simulink model "rayTrace_th"  (R2018b)
settings: Solver=FixedStepAuto  StartTime=0.0  StopTime=0  FixedStep=1  RelTol=1e-3
values from neighbouring files (symbols this model uses):
  grnd2CamRotMat = calculateRotationMatrix(     camEulAngles_rad(1),camEulAngles_rad(2),camEulAngles_rad(3))    [rayTrace_init.m]    (also in rayTrace_ts1.m = calculateRotationMatrix(     roll_deg*pi/180,pitch_deg*pi/18; rayTrace_ts3.m = calculateRotationMatrix(     roll_deg*pi/180,pitch_deg*pi/18; rayTrace_ts4.m)
  pixelCol = pixelCoords(ii,2)    [rayTrace_ts1.m]    (also in rayTrace_ts2.m; rayTrace_ts4.m = mean([pixCoords(2) pixCoords(4)]))
  pixelRow = pixelCoords(ii,1)    [rayTrace_ts1.m]    (also in rayTrace_ts2.m; rayTrace_ts4.m = mean([pixCoords(1) pixCoords(3)]))
undefined symbols (not defined in the file or in its folder): getVal, rayTrace, rayTrace_ul
settings Model: Creator=mcobb  LastModifiedBy=MAE-NCSUCORE

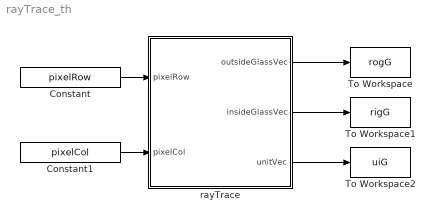
== system rayTrace_th ==
  Constant : Constant  Value=pixelRow
  Constant1 : Constant  Value=pixelCol
  To Workspace : ToWorkspace  VariableName=rogG  SampleTime=-1
  To Workspace1 : ToWorkspace  VariableName=rigG  SampleTime=-1
  To Workspace2 : ToWorkspace  VariableName=uiG  SampleTime=-1
  rayTrace : Subsystem  AncestorBlock=rayTrace_ul/rayTrace  mask{camPosVec_cm=[-30.5 -2 26], camEulAngles_deg=[0 133.9 180.6], dist2Glass_cm=7, indOfRefVec=[1 1 1], glassPlane=1, glassThickness_cm=0.75*2.54, imageDimsVec_px=getVal('sideImageSize_px'), camFOV_deg=getVal('cameraFOV_deg')}
      mask prompts: camPosVec_cm "Camera Position Vector, cm"; camEulAngles_deg "Camera Euler Angles, deg"; dist2Glass_cm "Distance to glass, cm"; indOfRefVec "Indices of refraction [air glass water]"; glassPlane "Glass plane (1 = xy, 2 = xz)"; glassThickness_cm "Glass thickness, cm"; imageDimsVec_px "Image dimensions, px [rows cols]"; camFOV_deg "Camera field of view angles,deg  [horiz vert]"
      mask init:
      | rayTrace_init
  wires:
  Constant/1 -> rayTrace/1(pixelRow)
  Constant1/1 -> rayTrace/2(pixelCol)
  rayTrace/1(outsideGlassVec) -> To Workspace/1
  rayTrace/3(unitVec) -> To Workspace2/1
  rayTrace/2(insideGlassVec) -> To Workspace1/1

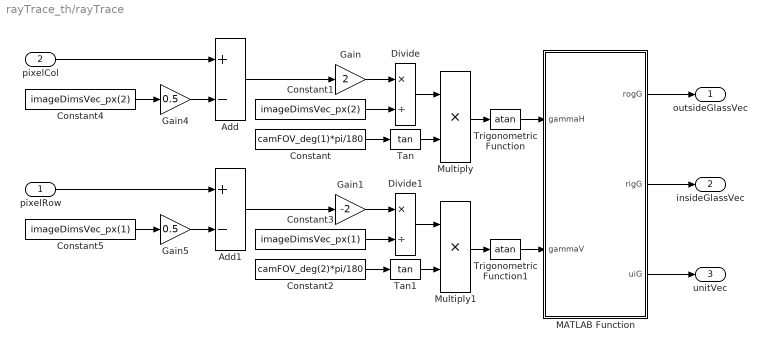
== system rayTrace_th/rayTrace ==
  pixelRow : Inport
  pixelCol : Inport  Port=2
  Add : Sum  Inputs=+-
  Add1 : Sum  Inputs=+-
  Constant : Constant  Value=camFOV_deg(1)*pi/180
  Constant1 : Constant  Value=imageDimsVec_px(2)
  Constant2 : Constant  Value=camFOV_deg(2)*pi/180
  Constant3 : Constant  Value=imageDimsVec_px(1)
  Constant4 : Constant  Value=imageDimsVec_px(2)
  Constant5 : Constant  Value=imageDimsVec_px(1)
  Divide : Product  Inputs=*/
  Divide1 : Product  Inputs=*/
  Gain : Gain  Gain=2
  Gain1 : Gain  Gain=-2
  Gain4 : Gain  Gain=0.5
  Gain5 : Gain  Gain=0.5
  MATLAB Function : MATLAB Function  TreatAsAtomicUnit=on
  Multiply : Product
  Multiply1 : Product
  Tan : Trigonometry  Operator=tan
  Tan1 : Trigonometry  Operator=tan
  Trigonometric Function : Trigonometry  Operator=atan
  Trigonometric Function1 : Trigonometry  Operator=atan
  outsideGlassVec : Outport
  insideGlassVec : Outport  Port=2
  unitVec : Outport  Port=3
  wires:
  Add1/1 -> Gain1/1
  Gain5/1 -> Add1/2
  pixelRow/1 -> Add1/1
  Constant5/1 -> Gain5/1
  Gain4/1 -> Add/2
  Constant4/1 -> Gain4/1
  Add/1 -> Gain/1
  pixelCol/1 -> Add/1
  Divide1/1 -> Multiply1/1
  Tan1/1 -> Multiply1/2
  Multiply1/1 -> Trigonometric Function1/1
  Trigonometric Function1/1 -> MATLAB Function/2(gammaV)
  Constant2/1 -> Tan1/1
  Constant3/1 -> Divide1/2
  Gain1/1 -> Divide1/1
  Constant1/1 -> Divide/2
  Gain/1 -> Divide/1
  Divide/1 -> Multiply/1
  Constant/1 -> Tan/1
  Tan/1 -> Multiply/2
  Multiply/1 -> Trigonometric Function/1
  Trigonometric Function/1 -> MATLAB Function/1(gammaH)
  MATLAB Function/1(rogG) -> outsideGlassVec/1
  MATLAB Function/3(uiG) -> unitVec/1
  MATLAB Function/2(rigG) -> insideGlassVec/1

== matlab function rayTrace_th/rayTrace/MATLAB Function ==
  data: rogG output; gammaH input; gammaV input; rigG output; uiG output; camPosVec_cm parameter; grnd2CamRotMat parameter; dist2Glass_cm parameter; indOfRefVec parameter; glassPlane parameter; glassThickness_cm parameter
function [rogG,rigG,uiG] = ...
    rayTrace(gammaH,gammaV,camPosVec_cm, grnd2CamRotMat, dist2Glass_cm, indOfRefVec,...
glassPlane, glassThickness_cm)

[rogG,rigG,uiG] = ...
    rayTrace(camPosVec_cm,grnd2CamRotMat,dist2Glass_cm,gammaH,gammaV,...
    indOfRefVec,glassPlane,glassThickness_cm);
